simulink model "Controller"  (R2018a)
settings: Solver=VariableStepAuto  StartTime=0.0  StopTime=10.0  RelTol=1e-3
settings Model: Creator=klukomski  LastModifiedBy=klukomski

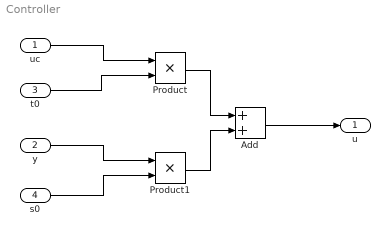
== system Controller ==
  uc : Inport
  y : Inport  Port=2
  t0 : Inport  Port=3
  s0 : Inport  Port=4
  Add : Sum
  Product : Product
  Product1 : Product
  u : Outport
  wires:
  Add/1 -> u/1
  Product/1 -> Add/1
  Product1/1 -> Add/2
  uc/1 -> Product/1
  y/1 -> Product1/1
  t0/1 -> Product/2
  s0/1 -> Product1/2
